simulink model "ProyectoProcesamiento1"  (R2015b)
settings: Solver=VariableStepAuto  StartTime=0.0  StopTime=10.0  RelTol=1e-3
libraries: simulink x2
settings Model: Creator=63942250  LastModifiedBy=63942250

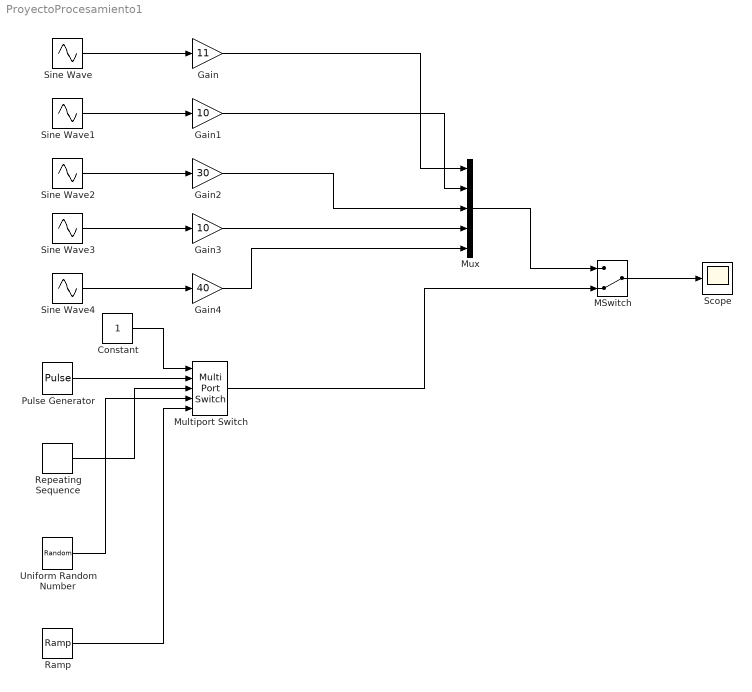
== system ProyectoProcesamiento1 ==
  Constant : Constant  VectorParams1D=off  LockScale=on
  Gain : Gain  Gain=11
  Gain1 : Gain  Gain=10
  Gain2 : Gain  Gain=30
  Gain3 : Gain  Gain=10
  Gain4 : Gain  Gain=40
  MSwitch : ManualSwitch  CurrentSetting=0
  Multiport Switch : MultiPortSwitch  Inputs=4
  Mux : Mux  Inputs=5
  Pulse Generator : DiscretePulseGenerator  PulseType=Time based  Amplitude=5  Period=10  PulseWidth=5
  Ramp : simulink/Sources/Ramp  slope=20  start=0  X0=0
  Repeating Sequence : simulink/Sources/Repeating Sequence  rep_seq_t=[0 2]  rep_seq_y=[0 2]
  Scope : Scope
  Sine Wave{,1..4} (5 alike) : Sin  SampleTime=0
  Uniform Random Number : UniformRandomNumber  SampleTime=0.1
  wires:
  Sine Wave/1 -> Gain/1
  Pulse Generator/1 -> Multiport Switch/2
  Multiport Switch/1 -> MSwitch/2
  Repeating Sequence/1 -> Multiport Switch/3
  Uniform Random Number/1 -> Multiport Switch/4
  Ramp/1 -> Multiport Switch/5
  Constant/1 -> Multiport Switch/1
  Sine Wave1/1 -> Gain1/1
  Sine Wave2/1 -> Gain2/1
  Sine Wave4/1 -> Gain4/1
  Sine Wave3/1 -> Gain3/1
  Gain4/1 -> Mux/5
  Gain3/1 -> Mux/4
  Gain2/1 -> Mux/3
  Gain1/1 -> Mux/2
  Gain/1 -> Mux/1
  Mux/1 -> MSwitch/1
  MSwitch/1 -> Scope/1
